simulink model "SM_differential"  (R2022b)
settings: Solver=ode4  StartTime=0.0  StopTime=10.0  FixedStep=0.01  RelTol=1e-3
settings Model: Creator=张倬境  LastModifiedBy=张倬境

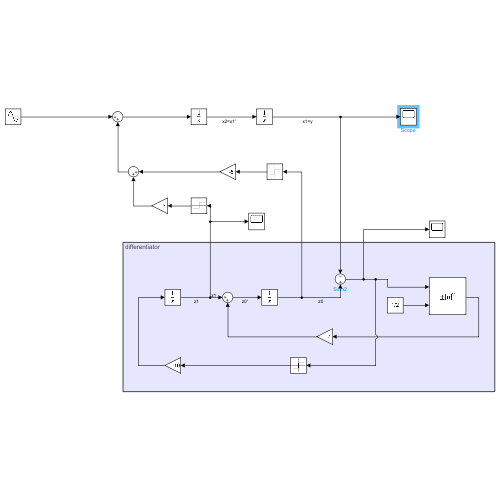
[thumbnail: Simulink's stored preview of the top-level diagram]
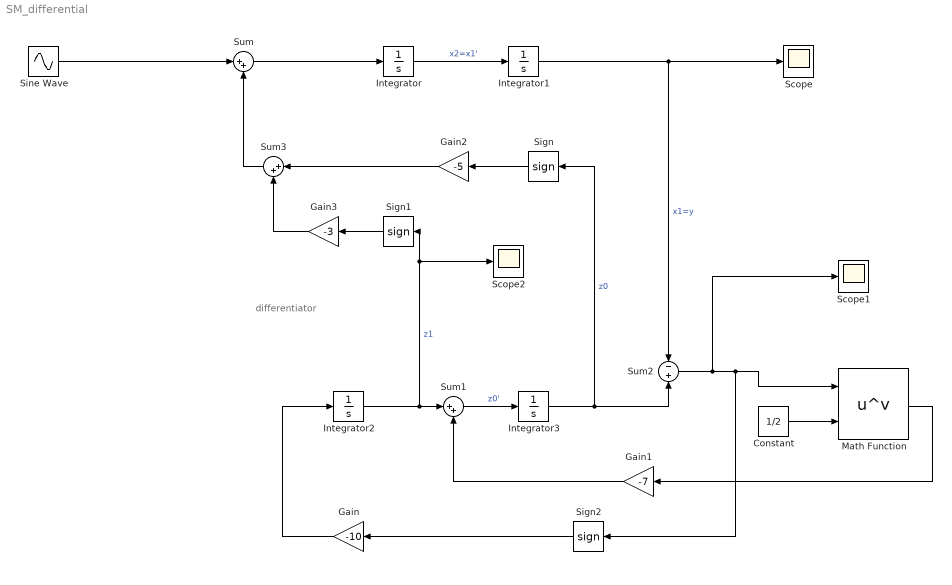
== system SM_differential ==
  note: differentiator
  Constant : Constant  Value=1/2
  Gain : Gain  Gain=-10
  Gain1 : Gain  Gain=-7
  Gain2 : Gain  Gain=-5
  Gain3 : Gain  Gain=-3
  Integrator{,1..3} (4 alike) : Integrator
  Math Function : Math  Operator=pow  SignedPower=on
  Scope : Scope
  Scope1 : Scope
  Scope2 : Scope
  Sign : Signum
  Sign1 : Signum
  Sign2 : Signum
  Sine Wave : Sin  SampleTime=0
  Sum : Sum  Inputs=|++
  Sum1 : Sum  Inputs=|++
  Sum2 : Sum  Inputs=-|+
  Sum3 : Sum  Inputs=|++
  wires:
  Integrator/1 -> Integrator1/1  "x2=x1'"
  Sum/1 -> Integrator/1
  Integrator1/1 -> Scope/1, Sum2/1  "x1=y"
  Integrator3/1 -> Sign/1, Sum2/2  "z0"
  Gain/1 -> Integrator2/1
  Sum1/1 -> Integrator3/1  "z0'"
  Constant/1 -> Math Function/2
  Sum2/1 -> Scope1/1, Sign2/1, Math Function/1
  Math Function/1 -> Gain1/1
  Gain1/1 -> Sum1/2
  Gain2/1 -> Sum3/1
  Sign/1 -> Gain2/1
  Sign1/1 -> Gain3/1
  Integrator2/1 -> Scope2/1, Sign1/1, Sum1/1  "z1"
  Gain3/1 -> Sum3/2
  Sum3/1 -> Sum/2
  Sign2/1 -> Gain/1
  Sine Wave/1 -> Sum/1
